simulink model "Quad_PID_attack_done"  (R2025a)
settings: Solver=ode4  StartTime=0.0  StopTime=40  FixedStep=0.001  RelTol=1e-3
undefined symbols (not defined in the file): DiscIntNeverNeededParam, Ts
libraries: simulink x6
settings Model: Creator=Qi  LastModifiedBy=shaoc
settings SolverCC: AlgebraicLoopSolver=TrustRegion
settings DataIOCC: ReturnWorkspaceOutputs=off
settings DebuggingCC: UnconnectedInputMsg=warning  UnconnectedOutputMsg=warning  UnconnectedLineMsg=warning  ArithmeticOperatorsInVariantConditions=warning
settings ModelReferenceCC: EnableRefExpFcnMdlSchedulingChecks=on
settings SFSimCC: CustomCodeUndefinedFunction=UseInterfaceOnly
settings RTWCC: GPUComputeCapability=3.5

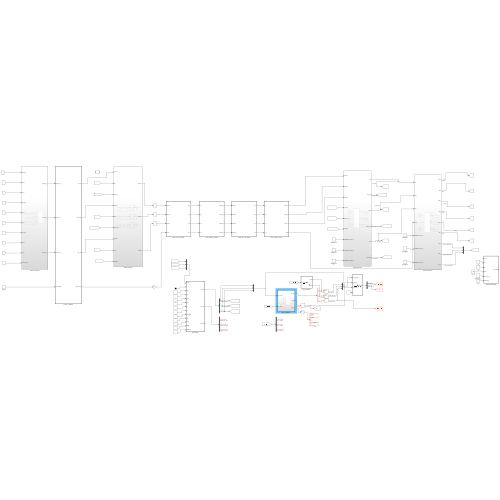
[thumbnail: Simulink's stored preview of the top-level diagram]
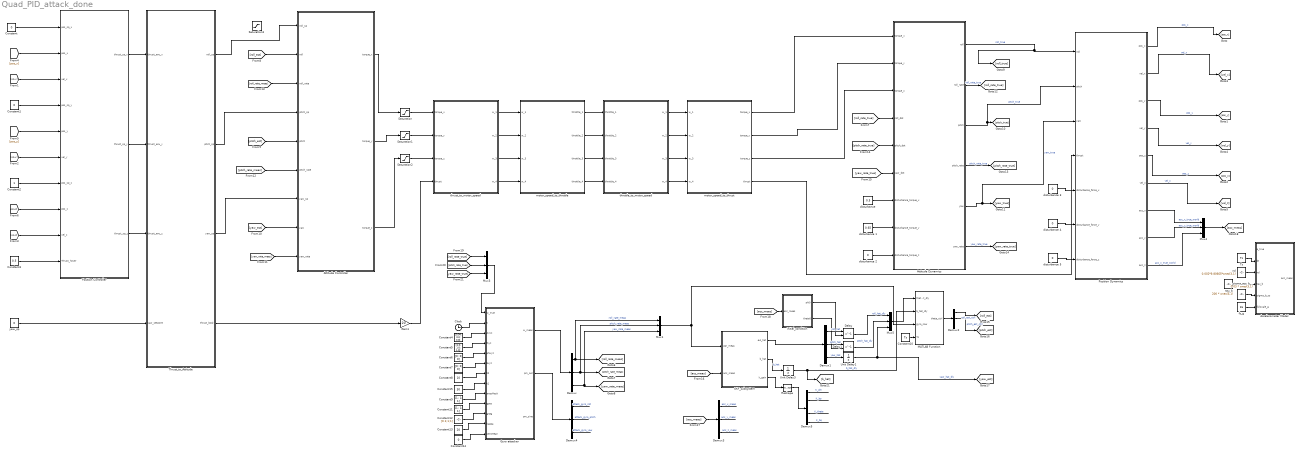
== system Quad_PID_attack_done ==
  Accelerometer Model : MATLAB Function  TreatAsAtomicUnit=on
  Attitude Controller : Subsystem
  Attitude Dynamics : Subsystem
  Clock : Clock
  Constant : Constant  Value=0
  Constant1 : Constant  Value=0
  Constant10 : Constant  Value=Ts  SampleTime=-1
  Constant11 : Constant  Value=[1; 1; 1]
  Constant12 : Constant  Value=[0.1;1;1]
  Constant13 : Constant  Value=20
  Constant14 : Constant  Value=0
  Constant15 : Constant  Value=30
  Constant2 : Constant
  Constant3 : Constant  Value=0.5
  Constant4 : Constant  Value=[0.04; 0.0; 0.0]
  Constant5 : Constant  Value=[1.0; 1.0; 1.0]
  Constant6 : Constant  Value=[0; 0; 0]
  Constant7 : Constant  Value=[0; 0; 0]
  Constant8 : Constant  Value=10
  Constant9 : Constant  Value=[1; 1; 1]
  Delay : Delay  DelayLength=1  InitialConditionSource=Input port  SampleTime=Ts
      settings: InputPortMap=u0,p4
  Delay1 : Delay  DelayLength=1  InitialConditionSource=Input port  SampleTime=Ts
      settings: InputPortMap=u0,p4
  Demux{,1..4} (5 alike) : Demux  Outputs=3
  Demux5 : Demux  Outputs=8
  EKF_subsystem : Subsystem  TreatAsAtomicUnit=on  SystemSampleTime=Ts
  Gain1 : Gain  Gain=20
  Gyro attacker : MATLAB Function  TreatAsAtomicUnit=on
  MATLAB Function : MATLAB Function  TreatAsAtomicUnit=on
  Mux{1,3..5} (4 alike) : Mux  Inputs=3
  Position Controller : Subsystem
  Position Dynamics : Subsystem
  Reshape : Reshape
  Saturation : Saturate  UpperLimit=1  LowerLimit=-1
  Saturation1 : Saturate  UpperLimit=1  LowerLimit=-1
  Saturation2 : Saturate  UpperLimit=1  LowerLimit=-1
  Saturation3 : Saturate  UpperLimit=10/180*pi  LowerLimit=-10/180*pi
  Thrust_to_Attitude : MATLAB Function  TreatAsAtomicUnit=on
  Ts : Constant  Value=Ts
  Unit Delay1 : UnitDelay  InitialCondition=true  SampleTime=Ts  HasFrameUpgradeWarning=on
  Unit Delay3 : UnitDelay  InitialCondition=true  SampleTime=Ts  HasFrameUpgradeWarning=on
  "disturbance " : Constant  Value=0.5
  disturbance 1 : Constant  Value=0.65
  disturbance {2..5} (4 alike) : Constant  Value=0
  "fs_g " : Constant  Value=16
  initial_condition : MATLAB Function  TreatAsAtomicUnit=on
  "motor_speed_to_throttle " : MATLAB Function  TreatAsAtomicUnit=on
  motor_speed_to_thrust : MATLAB Function  TreatAsAtomicUnit=on
  nd : Constant  Value=0.002*9.80665*ones(3,1)  VectorParams1D=off  LockScale=on
  sigma_acc_b : Constant  Value=0.03 * ones(3,1)  VectorParams1D=off  LockScale=on
  tau_b : Constant  Value=200 * ones(3,1)  VectorParams1D=off  LockScale=on
  throttle_to_motor_speed : MATLAB Function  TreatAsAtomicUnit=on
  thrust_to_motor_speed : MATLAB Function  TreatAsAtomicUnit=on
  yaw_sp : Constant  Value=0
  wires:
  yaw_sp/1 -> Thrust_to_Attitude/4(yaw_setpoint)
  Thrust_to_Attitude/4(thrust_body) -> Gain1/1
  Constant/1 -> Position Controller/1(pos_sp_x)
  [pos_x] -> Position Controller/2(pos_x)
  Constant1/1 -> Position Controller/4(pos_sp_y)
  [pos_z] -> Position Controller/8(pos_z)
  Constant2/1 -> Position Controller/7(pos_sp_z)
  Position Controller/1(thrust_sp_x) -> Thrust_to_Attitude/1(thrust_enu_x)
  Position Controller/2(thrust_sp_y) -> Thrust_to_Attitude/2(thrust_enu_y)
  Position Controller/3(thrust_sp_z) -> Thrust_to_Attitude/3(thrust_enu_z)
  [yaw_est] -> Attitude Controller/8(yaw)
  [roll_est] -> Attitude Controller/2(roll)
  [pitch_est] -> Attitude Controller/5(pitch)
  Thrust_to_Attitude/2(pitch_sp) -> Attitude Controller/4(pitch_sp)
  Thrust_to_Attitude/3(yaw_sp) -> Attitude Controller/7(yaw_sp)
  Attitude Controller/2(torque_y) -> Saturation1/1
  Attitude Controller/1(torque_x) -> Saturation/1
  Attitude Controller/3(torque_z) -> Saturation2/1
  [vel_x] -> Position Controller/3(vel_x)
  [pos_y] -> Position Controller/5(pos_y)
  [vel_y] -> Position Controller/6(vel_y)
  [vel_z] -> Position Controller/9(vel_z)
  [roll_rate_meas] -> Attitude Controller/3(roll_rate)
  [pitch_rate_meas] -> Attitude Controller/6(pitch_rate)
  [yaw_rate_meas] -> Attitude Controller/9(yaw_rate)
  Attitude Dynamics/3(pitch) -> Position Dynamics/2(pitch), [pitch_true]  "pitch_true"
  Attitude Dynamics/1(roll) -> [roll_true], Position Dynamics/1(roll)  "roll_true"
  Attitude Dynamics/5(yaw) -> [yaw_true], Position Dynamics/3(yaw)  "yaw_true"
  motor_speed_to_thrust/1(torque_x) -> Attitude Dynamics/1(torque_x)
  motor_speed_to_thrust/2(torque_y) -> Attitude Dynamics/2(torque_y)
  [roll_rate_true] -> Attitude Dynamics/4(roll_dot)
  motor_speed_to_thrust/3(torque_z) -> Attitude Dynamics/3(torque_z)
  [pitch_rate_true] -> Attitude Dynamics/5(pitch_dot)
  [yaw_rate_true] -> Attitude Dynamics/6(yaw_dot)
  Attitude Dynamics/2(roll_rate) -> [roll_rate_true]  "roll_rate_true"
  Attitude Dynamics/4(pitch_rate) -> [pitch_rate_true]  "pitch_rate_true"
  Attitude Dynamics/6(yaw_rate) -> [yaw_rate_true]  "yaw_rate_true"
  motor_speed_to_thrust/4(thrust) -> Position Dynamics/4(thrust)
  Position Dynamics/1(pos_x) -> [pos_x]  "pos_x"
  Position Dynamics/3(pos_y) -> [pos_y]  "pos_y"
  Position Dynamics/4(vel_y) -> [vel_y]  "vel_y"
  Position Dynamics/5(pos_z) -> [pos_z]  "pos_z"
  Position Dynamics/6(vel_z) -> [vel_z]  "vel_z"
  Constant3/1 -> Position Controller/10(Thrust_hover)
  disturbance 2/1 -> Attitude Dynamics/9(disturbance_torque_z)
  disturbance 1/1 -> Attitude Dynamics/8(disturbance_torque_y)
  "disturbance "/1 -> Attitude Dynamics/7(disturbance_torque_x)
  disturbance 3/1 -> Position Dynamics/5(disturbance_force_x)
  disturbance 4/1 -> Position Dynamics/6(disturbance_force_y)
  disturbance 5/1 -> Position Dynamics/7(disturbance_force_z)
  thrust_to_motor_speed/1(w_1) -> "motor_speed_to_throttle "/1(w_1)
  thrust_to_motor_speed/3(w_3) -> "motor_speed_to_throttle "/3(w_3)
  thrust_to_motor_speed/4(w_4) -> "motor_speed_to_throttle "/4(w_4)
  thrust_to_motor_speed/2(w_2) -> "motor_speed_to_throttle "/2(w_2)
  "motor_speed_to_throttle "/1(throttle_1) -> throttle_to_motor_speed/1(throttle_1)
  "motor_speed_to_throttle "/2(throttle_2) -> throttle_to_motor_speed/2(throttle_2)
  "motor_speed_to_throttle "/3(throttle_3) -> throttle_to_motor_speed/3(throttle_3)
  "motor_speed_to_throttle "/4(throttle_4) -> throttle_to_motor_speed/4(throttle_4)
  throttle_to_motor_speed/1(w_1) -> motor_speed_to_thrust/1(w_1)
  throttle_to_motor_speed/2(w_2) -> motor_speed_to_thrust/2(w_2)
  throttle_to_motor_speed/3(w_3) -> motor_speed_to_thrust/3(w_3)
  throttle_to_motor_speed/4(w_4) -> motor_speed_to_thrust/4(w_4)
  Gain1/1 -> thrust_to_motor_speed/4(thrust)
  Position Dynamics/2(vel_x) -> [vel_x]  "vel_x"
  Saturation/1 -> thrust_to_motor_speed/1(torque_x)
  Saturation1/1 -> thrust_to_motor_speed/2(torque_y)
  Saturation2/1 -> thrust_to_motor_speed/3(torque_z)
  Clock/1 -> Gyro attacker/2(t)
  Constant4/1 -> Gyro attacker/3(Axyz)
  Constant5/1 -> Gyro attacker/4(fxyz)
  Constant6/1 -> Gyro attacker/5(phixyz)
  Constant7/1 -> Gyro attacker/6(bxyz)
  Constant8/1 -> Gyro attacker/7(t0)
  Constant9/1 -> Gyro attacker/9(axesMask)
  Gyro attacker/1(w_meas) -> Demux/1
  Demux/1 -> Mux1/1, [roll_rate_meas]  "roll_rate_meas"
  Demux/2 -> Mux1/2, [pitch_rate_meas]  "pitch_rate_meas"
  Demux/3 -> Mux1/3, [yaw_rate_meas]  "yaw_rate_meas"
  Position Dynamics/7(acc_x) -> Mux4/1  "acc_x_true_world"
  Position Dynamics/8(acc_y) -> Mux4/2  "acc_y_true_world"
  Position Dynamics/9(acc_z) -> Mux4/3  "acc_z_true_world"
  [roll_rate_true] -> Mux3/1
  [pitch_rate_true] -> Mux3/2
  [yaw_rate_true] -> Mux3/3
  Mux3/1 -> Gyro attacker/1(w_true)
  Mux1/1 -> MATLAB Function/3(gyro_now), EKF_subsystem/1(pqr_meas)
  EKF_subsystem/1(eul_hat) -> Demux1/1
  Demux1/1 -> Delay/1  "roll_hat"
  Delay/1 -> Mux5/1  "roll_hat_dly"
  Demux1/2 -> Delay1/1  "pitch_hat"
  Delay1/1 -> Mux5/2  "pitch_hat_dly"
  Demux1/3 -> Unit Delay1/1  "yaw_hat"
  Unit Delay1/1 -> Mux5/3, [yaw_est]  "yaw_hat_dly"
  EKF_subsystem/2(b_hat) -> Unit Delay3/1  "b_hat"
  Unit Delay3/1 -> MATLAB Function/2(b_hat_dly), [b_hat]  "b_hat_dly"
  Mux5/1 -> MATLAB Function/1(theta_hat_dly)
  Constant10/1 -> MATLAB Function/4(Ts)
  MATLAB Function/1(theta_ctrl) -> Demux2/1
  Demux2/1 -> [roll_est]  "roll_est_ctrl"
  Demux2/2 -> [pitch_est]  "pitch_est_ctrl"
  [acc_meas] -> EKF_subsystem/2(acc_meas)
  [acc_meas] -> Demux3/1
  Demux3/1 -> ?  "acc_x_meas"
  Demux3/2 -> ?  "acc_y_meas"
  Demux3/3 -> ?  "acc_z_meas"
  [acc_meas] -> initial_condition/1(acc_meas)
  initial_condition/1(phi0) -> Delay/2
  initial_condition/2(theta0) -> Delay1/2
  Ts/1 -> Accelerometer Model/2(dt)
  "fs_g "/1 -> Accelerometer Model/6(fullscale_g)
  nd/1 -> Accelerometer Model/3(nd)
  tau_b/1 -> Accelerometer Model/4(tau_b)
  sigma_acc_b/1 -> Accelerometer Model/5(sigma_b_ss)
  Mux4/1 -> [acc_meas]
  Demux4/3 -> ?  "attack_gyro_yaw"
  Demux4/1 -> ?  "attack_gyro_roll"
  Gyro attacker/2(pm_out) -> Demux4/1
  Demux4/2 -> ?  "attack_gyro_pitch"
  Constant11/1 -> Gyro attacker/10(gpos)
  Constant12/1 -> Gyro attacker/11(gneg)
  Constant13/1 -> Gyro attacker/12(kappa)
  Constant14/1 -> Gyro attacker/13(zeroMean)
  Constant15/1 -> Gyro attacker/8(t1)
  EKF_subsystem/3(k_gain) -> Reshape/1
  Reshape/1 -> Demux5/1
  Demux5/1 -> ?  "K_phi"
  Demux5/3 -> ?  "K_bp"
  Demux5/6 -> ?  "K_theta"
  Demux5/8 -> ?  "K_bq"
  Thrust_to_Attitude/1(roll_sp) -> Attitude Controller/1(roll_sp)

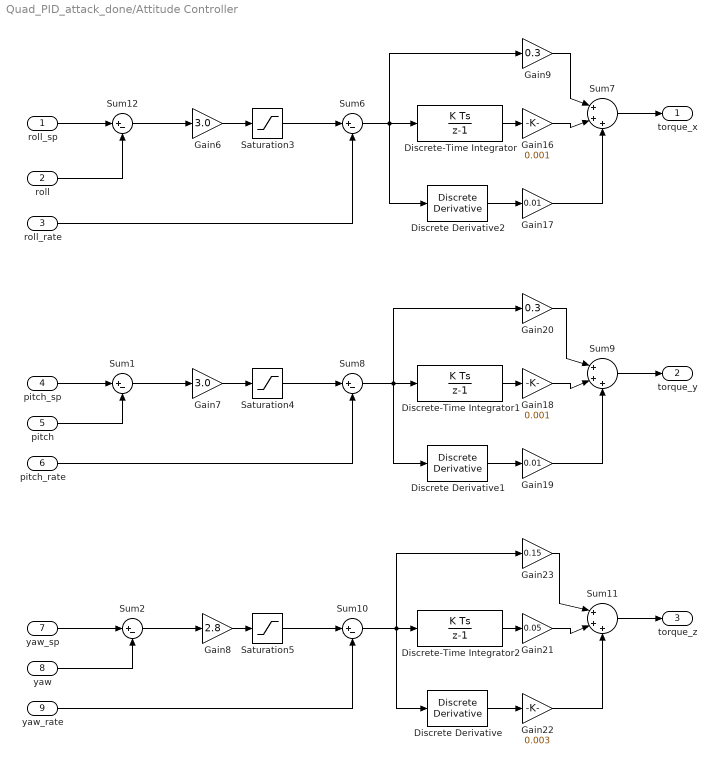
== system Quad_PID_attack_done/Attitude Controller ==
  roll_sp : Inport
  roll : Inport  Port=2
  roll_rate : Inport  Port=3
  pitch_sp : Inport  Port=4
  pitch : Inport  Port=5
  pitch_rate : Inport  Port=6
  yaw_sp : Inport  Port=7
  yaw : Inport  Port=8
  yaw_rate : Inport  Port=9
  Discrete Derivative : simulink/Discrete/Discrete Derivative  gainval=1.0  ICPrevScaledInput=0.0  OutMin=[]  OutMax=[]  OutDataType=fixdt(1, 16)  OutScaling=2^-10  DoSatur=off
  Discrete Derivative1 : simulink/Discrete/Discrete Derivative  gainval=1.0  ICPrevScaledInput=0.0  OutMin=[]  OutMax=[]  OutDataType=fixdt(1, 16)  OutScaling=2^-10  DoSatur=off
  Discrete Derivative2 : simulink/Discrete/Discrete Derivative  gainval=1.0  ICPrevScaledInput=0.0  OutMin=[]  OutMax=[]  OutDataType=fixdt(1, 16)  OutScaling=2^-10  DoSatur=off
  Discrete-Time Integrator : DiscreteIntegrator  SampleTime=-1  LimitOutput=on  UpperSaturationLimit=0.3  LowerSaturationLimit=-0.3  ICPrevOutput=DiscIntNeverNeededParam  ICPrevScaledInput=DiscIntNeverNeededParam
  Discrete-Time Integrator1 : DiscreteIntegrator  SampleTime=-1  LimitOutput=on  UpperSaturationLimit=0.3  LowerSaturationLimit=-0.3  ICPrevOutput=DiscIntNeverNeededParam  ICPrevScaledInput=DiscIntNeverNeededParam
  Discrete-Time Integrator2 : DiscreteIntegrator  SampleTime=-1  LimitOutput=on  UpperSaturationLimit=0.3  LowerSaturationLimit=-0.3  ICPrevOutput=DiscIntNeverNeededParam  ICPrevScaledInput=DiscIntNeverNeededParam
  Gain16 : Gain  Gain=0.001
  Gain17 : Gain  Gain=0.01
  Gain18 : Gain  Gain=0.001
  Gain19 : Gain  Gain=0.01
  Gain20 : Gain  Gain=0.3
  Gain21 : Gain  Gain=0.05
  Gain22 : Gain  Gain=0.003
  Gain23 : Gain  Gain=0.15
  Gain6 : Gain  Gain=3.0
  Gain7 : Gain  Gain=3.0
  Gain8 : Gain  Gain=2.8
  Gain9 : Gain  Gain=0.3
  Saturation3 : Saturate  UpperLimit=220/180*pi  LowerLimit=-220/180*pi
  Saturation4 : Saturate  UpperLimit=220/180*pi  LowerLimit=-220/180*pi
  Saturation5 : Saturate  UpperLimit=220/180*pi  LowerLimit=-220/180*pi
  Sum{1..2,6,8,10,12} (6 alike) : Sum  Inputs=|+-
  Sum11 : Sum  Inputs=|+++
  Sum7 : Sum  Inputs=|+++
  Sum9 : Sum  Inputs=|+++
  torque_x : Outport  VectorParamsAs1DForOutWhenUnconnected=off
  torque_y : Outport  Port=2  VectorParamsAs1DForOutWhenUnconnected=off
  torque_z : Outport  Port=3  VectorParamsAs1DForOutWhenUnconnected=off
  wires:
  Gain8/1 -> Saturation5/1
  Sum10/1 -> Discrete-Time Integrator2/1, Discrete Derivative/1, Gain23/1
  Sum6/1 -> Discrete-Time Integrator/1, Discrete Derivative2/1, Gain9/1
  Saturation4/1 -> Sum8/1
  Sum7/1 -> torque_x/1
  Discrete-Time Integrator2/1 -> Gain21/1
  Gain16/1 -> Sum7/2
  Sum8/1 -> Discrete-Time Integrator1/1, Discrete Derivative1/1, Gain20/1
  yaw_rate/1 -> Sum10/2
  Saturation5/1 -> Sum10/1
  Gain23/1 -> Sum11/1
  Saturation3/1 -> Sum6/1
  Discrete Derivative1/1 -> Gain19/1
  Gain17/1 -> Sum7/3
  Gain19/1 -> Sum9/3
  Gain22/1 -> Sum11/3
  Discrete Derivative/1 -> Gain22/1
  Gain7/1 -> Saturation4/1
  Discrete-Time Integrator1/1 -> Gain18/1
  Gain18/1 -> Sum9/2
  Gain9/1 -> Sum7/1
  Gain20/1 -> Sum9/1
  Discrete-Time Integrator/1 -> Gain16/1
  roll_rate/1 -> Sum6/2
  Sum9/1 -> torque_y/1
  Discrete Derivative2/1 -> Gain17/1
  Gain21/1 -> Sum11/2
  Gain6/1 -> Saturation3/1
  Sum11/1 -> torque_z/1
  pitch_rate/1 -> Sum8/2
  yaw/1 -> Sum2/2
  Sum1/1 -> Gain7/1
  roll_sp/1 -> Sum12/1
  pitch/1 -> Sum1/2
  Sum2/1 -> Gain8/1
  pitch_sp/1 -> Sum1/1
  roll/1 -> Sum12/2
  yaw_sp/1 -> Sum2/1
  Sum12/1 -> Gain6/1

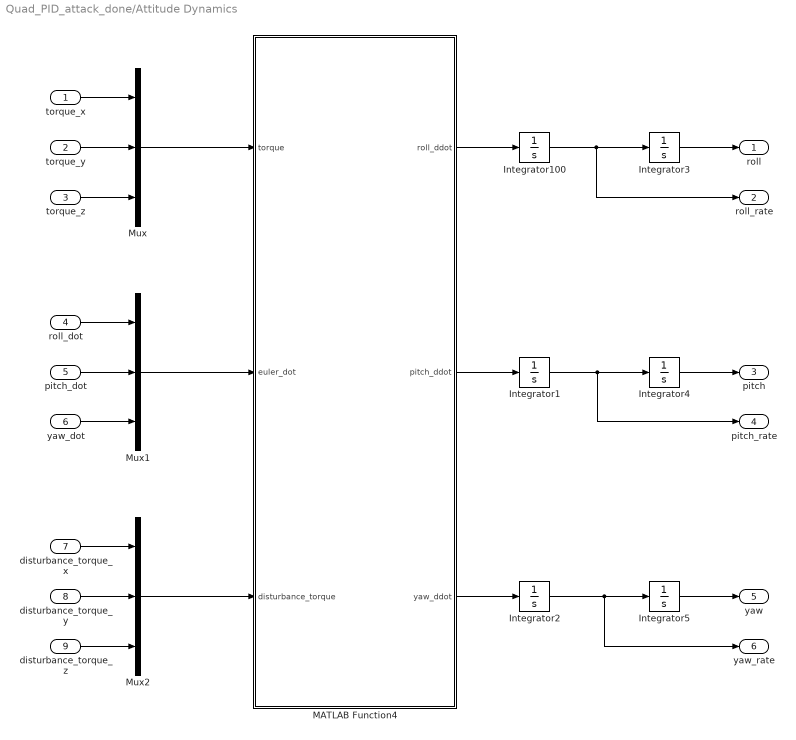
== system Quad_PID_attack_done/Attitude Dynamics ==
  torque_x : Inport
  torque_y : Inport  Port=2
  torque_z : Inport  Port=3
  roll_dot : Inport  Port=4
  pitch_dot : Inport  Port=5
  yaw_dot : Inport  Port=6
  disturbance_torque_x : Inport  Port=7
  disturbance_torque_y : Inport  Port=8
  disturbance_torque_z : Inport  Port=9
  Integrator{1..5,100} (6 alike) : Integrator
  MATLAB Function4 : MATLAB Function  TreatAsAtomicUnit=on
  Mux : Mux  Inputs=3
  Mux1 : Mux  Inputs=3
  Mux2 : Mux  Inputs=3
  roll : Outport  VectorParamsAs1DForOutWhenUnconnected=off
  roll_rate : Outport  Port=2  VectorParamsAs1DForOutWhenUnconnected=off
  pitch : Outport  Port=3  VectorParamsAs1DForOutWhenUnconnected=off
  pitch_rate : Outport  Port=4  VectorParamsAs1DForOutWhenUnconnected=off
  yaw : Outport  Port=5  VectorParamsAs1DForOutWhenUnconnected=off
  yaw_rate : Outport  Port=6  VectorParamsAs1DForOutWhenUnconnected=off
  wires:
  Integrator100/1 -> roll_rate/1, Integrator3/1
  Integrator4/1 -> pitch/1
  MATLAB Function4/3(yaw_ddot) -> Integrator2/1
  Integrator3/1 -> roll/1
  Integrator1/1 -> pitch_rate/1, Integrator4/1
  Integrator2/1 -> yaw_rate/1, Integrator5/1
  MATLAB Function4/1(roll_ddot) -> Integrator100/1
  MATLAB Function4/2(pitch_ddot) -> Integrator1/1
  Integrator5/1 -> yaw/1
  disturbance_torque_y/1 -> Mux2/2
  disturbance_torque_z/1 -> Mux2/3
  disturbance_torque_x/1 -> Mux2/1
  Mux2/1 -> MATLAB Function4/3(disturbance_torque)
  yaw_dot/1 -> Mux1/3
  pitch_dot/1 -> Mux1/2
  roll_dot/1 -> Mux1/1
  Mux1/1 -> MATLAB Function4/2(euler_dot)
  torque_y/1 -> Mux/2
  torque_z/1 -> Mux/3
  torque_x/1 -> Mux/1
  Mux/1 -> MATLAB Function4/1(torque)

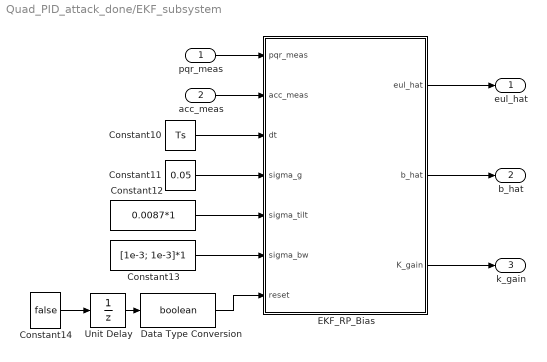
== system Quad_PID_attack_done/EKF_subsystem ==
  pqr_meas : Inport
  acc_meas : Inport  Port=2
  Constant10 : Constant  Value=Ts  SampleTime=-1
  Constant11 : Constant  Value=0.05
  Constant12 : Constant  Value=0.0087*1
  Constant13 : Constant  Value=[1e-3; 1e-3]*1
  Constant14 : Constant  Value=false
  Data Type Conversion : DataTypeConversion  OutDataTypeStr=boolean  SaturateOnIntegerOverflow=off  RndMeth=Floor
  EKF_RP_Bias : MATLAB Function  TreatAsAtomicUnit=on
  Unit Delay : UnitDelay  InitialCondition=true  SampleTime=Ts  HasFrameUpgradeWarning=on
  eul_hat : Outport  VectorParamsAs1DForOutWhenUnconnected=off
  b_hat : Outport  Port=2  VectorParamsAs1DForOutWhenUnconnected=off
  k_gain : Outport  Port=3  VectorParamsAs1DForOutWhenUnconnected=off
  wires:
  Unit Delay/1 -> Data Type Conversion/1
  Constant14/1 -> Unit Delay/1
  Constant11/1 -> EKF_RP_Bias/4(sigma_g)
  Constant10/1 -> EKF_RP_Bias/3(dt)
  Data Type Conversion/1 -> EKF_RP_Bias/7(reset)
  Constant13/1 -> EKF_RP_Bias/6(sigma_bw)
  Constant12/1 -> EKF_RP_Bias/5(sigma_tilt)
  EKF_RP_Bias/1(eul_hat) -> eul_hat/1
  EKF_RP_Bias/2(b_hat) -> b_hat/1
  pqr_meas/1 -> EKF_RP_Bias/1(pqr_meas)
  acc_meas/1 -> EKF_RP_Bias/2(acc_meas)
  EKF_RP_Bias/3(K_gain) -> k_gain/1

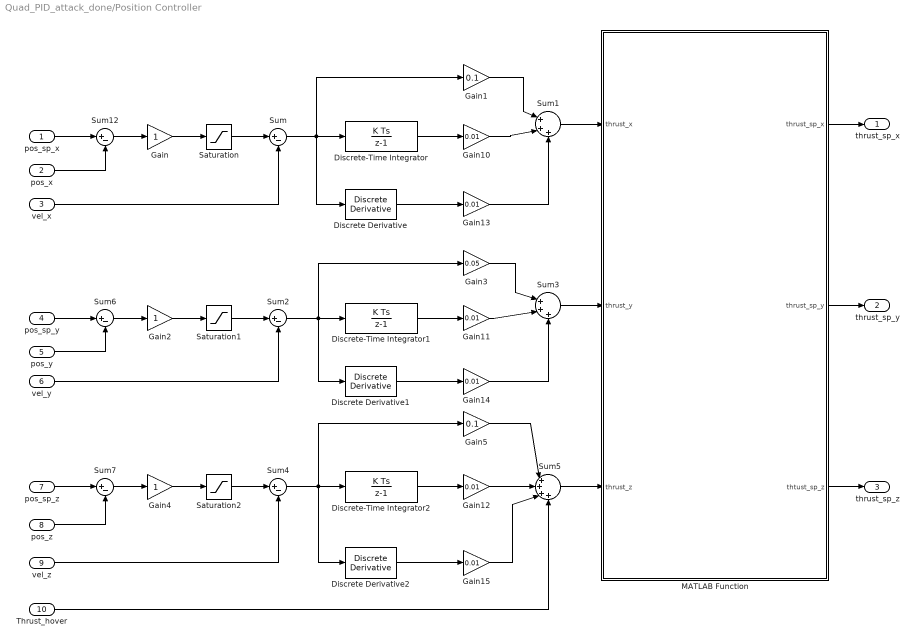
== system Quad_PID_attack_done/Position Controller ==
  pos_sp_x : Inport
  pos_x : Inport  Port=2
  vel_x : Inport  Port=3
  pos_sp_y : Inport  Port=4
  pos_y : Inport  Port=5
  vel_y : Inport  Port=6
  pos_sp_z : Inport  Port=7
  pos_z : Inport  Port=8
  vel_z : Inport  Port=9
  Thrust_hover : Inport  Port=10
  Discrete Derivative : simulink/Discrete/Discrete Derivative  gainval=1.0  ICPrevScaledInput=0.0  OutMin=[]  OutMax=[]  OutDataType=fixdt(1, 16)  OutScaling=2^-10  DoSatur=off
  Discrete Derivative1 : simulink/Discrete/Discrete Derivative  gainval=1.0  ICPrevScaledInput=0.0  OutMin=[]  OutMax=[]  OutDataType=fixdt(1, 16)  OutScaling=2^-10  DoSatur=off
  Discrete Derivative2 : simulink/Discrete/Discrete Derivative  gainval=1.0  ICPrevScaledInput=0.0  OutMin=[]  OutMax=[]  OutDataType=fixdt(1, 16)  OutScaling=2^-10  DoSatur=off
  Discrete-Time Integrator : DiscreteIntegrator  SampleTime=-1  LimitOutput=on  UpperSaturationLimit=0.9  LowerSaturationLimit=-0.9  ICPrevOutput=DiscIntNeverNeededParam  ICPrevScaledInput=DiscIntNeverNeededParam
  Discrete-Time Integrator1 : DiscreteIntegrator  SampleTime=-1  LimitOutput=on  UpperSaturationLimit=0.9  LowerSaturationLimit=-0.9  ICPrevOutput=DiscIntNeverNeededParam  ICPrevScaledInput=DiscIntNeverNeededParam
  Discrete-Time Integrator2 : DiscreteIntegrator  SampleTime=-1  LimitOutput=on  UpperSaturationLimit=0.9  LowerSaturationLimit=-0.9  ICPrevOutput=DiscIntNeverNeededParam  ICPrevScaledInput=DiscIntNeverNeededParam
  Gain : Gain
  Gain1 : Gain  Gain=0.1
  Gain{10..15} (6 alike) : Gain  Gain=0.01
  Gain2 : Gain
  Gain3 : Gain  Gain=0.05
  Gain4 : Gain
  Gain5 : Gain  Gain=0.1
  MATLAB Function : MATLAB Function  TreatAsAtomicUnit=on
  Saturation : Saturate  UpperLimit=5  LowerLimit=-5
  Saturation1 : Saturate  UpperLimit=5  LowerLimit=-5
  Saturation2 : Saturate  UpperLimit=2  LowerLimit=-2
  Sum{,2,4,6..7,12} (6 alike) : Sum  Inputs=|+-
  Sum1 : Sum  Inputs=|+++
  Sum3 : Sum  Inputs=|+++
  Sum5 : Sum  Inputs=|++++
  thrust_sp_x : Outport  VectorParamsAs1DForOutWhenUnconnected=off
  thrust_sp_y : Outport  Port=2  VectorParamsAs1DForOutWhenUnconnected=off
  thrust_sp_z : Outport  Port=3  VectorParamsAs1DForOutWhenUnconnected=off
  wires:
  Gain4/1 -> Saturation2/1
  Saturation1/1 -> Sum2/1
  MATLAB Function/1(thrust_sp_x) -> thrust_sp_x/1
  vel_x/1 -> Sum/2
  Gain/1 -> Saturation/1
  Gain11/1 -> Sum3/2
  Sum2/1 -> Discrete-Time Integrator1/1, Discrete Derivative1/1, Gain3/1
  Gain3/1 -> Sum3/1
  Sum4/1 -> Discrete-Time Integrator2/1, Discrete Derivative2/1, Gain5/1
  vel_z/1 -> Sum4/2
  Gain2/1 -> Saturation1/1
  Sum5/1 -> MATLAB Function/3(thrust_z)
  Discrete Derivative2/1 -> Gain15/1
  Saturation2/1 -> Sum4/1
  Discrete-Time Integrator/1 -> Gain10/1
  MATLAB Function/2(thrust_sp_y) -> thrust_sp_y/1
  MATLAB Function/3(thtust_sp_z) -> thrust_sp_z/1
  Saturation/1 -> Sum/1
  Gain1/1 -> Sum1/1
  Sum1/1 -> MATLAB Function/1(thrust_x)
  Gain13/1 -> Sum1/3
  Sum/1 -> Discrete-Time Integrator/1, Discrete Derivative/1, Gain1/1
  Discrete Derivative1/1 -> Gain14/1
  Discrete Derivative/1 -> Gain13/1
  Discrete-Time Integrator2/1 -> Gain12/1
  Discrete-Time Integrator1/1 -> Gain11/1
  Thrust_hover/1 -> Sum5/4
  Gain5/1 -> Sum5/1
  Sum3/1 -> MATLAB Function/2(thrust_y)
  Gain12/1 -> Sum5/2
  Gain15/1 -> Sum5/3
  Gain14/1 -> Sum3/3
  vel_y/1 -> Sum2/2
  pos_sp_x/1 -> Sum12/1
  Sum12/1 -> Gain/1
  pos_x/1 -> Sum12/2
  pos_sp_z/1 -> Sum7/1
  Sum7/1 -> Gain4/1
  pos_z/1 -> Sum7/2
  pos_y/1 -> Sum6/2
  Sum6/1 -> Gain2/1
  pos_sp_y/1 -> Sum6/1
  Gain10/1 -> Sum1/2

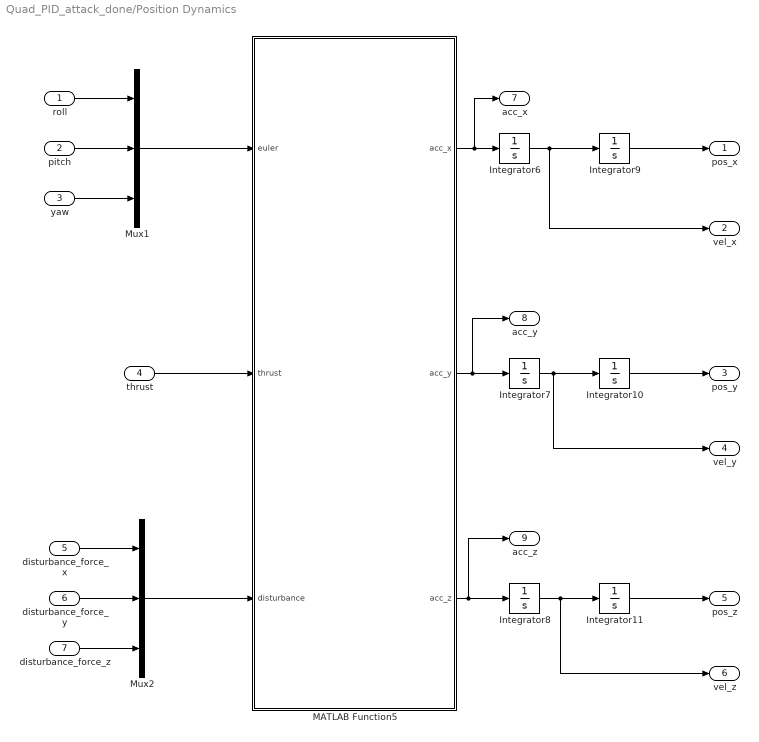
== system Quad_PID_attack_done/Position Dynamics ==
  roll : Inport
  pitch : Inport  Port=2
  yaw : Inport  Port=3
  thrust : Inport  Port=4
  disturbance_force_x : Inport  Port=5
  disturbance_force_y : Inport  Port=6
  disturbance_force_z : Inport  Port=7
  Integrator{6..11} (6 alike) : Integrator
  MATLAB Function5 : MATLAB Function  TreatAsAtomicUnit=on
  Mux1 : Mux  Inputs=3
  Mux2 : Mux  Inputs=3
  pos_x : Outport  VectorParamsAs1DForOutWhenUnconnected=off
  vel_x : Outport  Port=2  VectorParamsAs1DForOutWhenUnconnected=off
  pos_y : Outport  Port=3  VectorParamsAs1DForOutWhenUnconnected=off
  vel_y : Outport  Port=4  VectorParamsAs1DForOutWhenUnconnected=off
  pos_z : Outport  Port=5  VectorParamsAs1DForOutWhenUnconnected=off
  vel_z : Outport  Port=6  VectorParamsAs1DForOutWhenUnconnected=off
  acc_x : Outport  Port=7  VectorParamsAs1DForOutWhenUnconnected=off
  acc_y : Outport  Port=8  VectorParamsAs1DForOutWhenUnconnected=off
  acc_z : Outport  Port=9  VectorParamsAs1DForOutWhenUnconnected=off
  wires:
  Integrator7/1 -> vel_y/1, Integrator10/1
  MATLAB Function5/1(acc_x) -> acc_x/1, Integrator6/1
  MATLAB Function5/3(acc_z) -> acc_z/1, Integrator8/1
  Integrator6/1 -> vel_x/1, Integrator9/1
  MATLAB Function5/2(acc_y) -> acc_y/1, Integrator7/1
  thrust/1 -> MATLAB Function5/2(thrust)
  Integrator8/1 -> vel_z/1, Integrator11/1
  Integrator9/1 -> pos_x/1
  Integrator10/1 -> pos_y/1
  Integrator11/1 -> pos_z/1
  roll/1 -> Mux1/1
  pitch/1 -> Mux1/2
  Mux1/1 -> MATLAB Function5/1(euler)
  yaw/1 -> Mux1/3
  disturbance_force_x/1 -> Mux2/1
  disturbance_force_z/1 -> Mux2/3
  Mux2/1 -> MATLAB Function5/3(disturbance)
  disturbance_force_y/1 -> Mux2/2

== matlab function Quad_PID_attack_done/motor_speed_to_throttle  ==
  data: w_1 input; throttle_1 output; w_2 input; w_3 input; w_4 input; throttle_2 output; throttle_3 output; throttle_4 output
function [throttle_1, throttle_2, throttle_3, throttle_4] = motor_speed_to_throttle(w_1, w_2, w_3, w_4)
    %%注意转速单位 rad/s or rpm 转/分   
    k_est = 718.07;
    d_est = 88.448;
    
    throttle_1 = (w_1 - d_est)/k_est;
    throttle_2 = (w_2 - d_est)/k_est;
    throttle_3 = (w_3 - d_est)/k_est;
    throttle_4 = (w_4 - d_est)/k_est;
end

== matlab function Quad_PID_attack_done/throttle_to_motor_speed ==
  data: throttle_1 input; w_1 output; throttle_2 input; throttle_3 input; throttle_4 input; w_2 output; w_3 output; w_4 output
function [w_1, w_2, w_3, w_4] = throttle_tomotor_speed(throttle_1, throttle_2, throttle_3, throttle_4)
    k = 718.07;
    d = 88.448;
    
    w_1 = k * throttle_1 + d;
    w_2 = k * throttle_2 + d;
    w_3 = k * throttle_3 + d;
    w_4 = k * throttle_4 + d;
end

== matlab function Quad_PID_attack_done/motor_speed_to_thrust ==
  data: torque_x output; w_1 input; w_2 input; torque_y output; w_3 input; w_4 input; torque_z output; thrust output
function [torque_x, torque_y, torque_z, thrust] = thrust_to_motor_speed(w_1, w_2, w_3, w_4)

d  = 0.2;
cT = 1.239e-5;
cM = 1.982e-7;


M4 = [-sqrt(2)/2*d*cT,sqrt(2)/2*d*cT,sqrt(2)/2*d*cT,-sqrt(2)/2*d*cT;
       sqrt(2)/2*d*cT,-sqrt(2)/2*d*cT,sqrt(2)/2*d*cT,-sqrt(2)/2*d*cT;
       cM,cM,-cM,-cM;
       cT,cT,cT,cT;];
   
u = M4 * [w_1^2 ;w_2^2 ;w_3^2 ;w_4^2];  

torque_x = u(1);
torque_y = u(2);
torque_z = u(3);
thrust   = u(4);


end

== matlab function Quad_PID_attack_done/Gyro attacker ==
  data: w_true input double size=[3 1]; w_meas output double size=[3 1]; t input double size=[1 1]; Axyz input double size=[3 1]; fxyz input double size=[3 1]; phixyz input double size=[3 1]; bxyz input double size=[3 1]; t0 input double size=[1 1]; t1 input; axesMask input double size=[3 1]; pm_out output; gpos input; gneg input; kappa input; zeroMean input; pm_sine output
function [w_meas, pm_out, pm_sine] = gyro_attack_asym_smooth_stateless( ...
    w_true, t, Axyz, fxyz, phixyz, bxyz, t0, t1, axesMask, ...
    gpos, gneg, kappa, zeroMean)
%#codegen
% Smooth (differentiable) asymmetric sine attack WITHOUT persistent state.
% Attack (including bias) is ON only for t0 <= t < t1. Outside: no attack.

% ---- ensure 3x1 columns ----
w_true   = reshape(w_true,   3,1);
Axyz     = reshape(Axyz,     3,1);
fxyz     = reshape(fxyz,     3,1);
phixyz   = reshape(phixyz,   3,1);
bxyz     = reshape(bxyz,     3,1);
axesMask = reshape(axesMask, 3,1);
gpos     = reshape(gpos,     3,1);
gneg     = reshape(gneg,     3,1);

% ---- timing, mask, enable-window ----
win   = double( (t >= t0) && (t < t1) );   % <-- NEW: window gate
t_eff = max(t - t0, 0);                    % time since start (phase continuity)
mask  = double(axesMask ~= 0);

% ---- base sine ----
arg = 2*pi.*fxyz.*t_eff + phixyz;
s   = sin(arg);

% ---- smooth gate & shaping (C^inf) ----
H        = 0.5 * (1 + tanh(kappa * s));       % 0..1 smoothly across s=0
gain_s   = gneg + (gpos - gneg) .* H;         % per-axis, smooth
s_shaped = gain_s .* s;                       % unitless

% ---- optional analytic DC removal (approx) ----
% Hard half-wave has mean (gpos-gneg)/pi; for smooth gate this is close.
if zeroMean ~= 0
    s_shaped = s_shaped - (gpos - gneg)/pi;
end

% ---- scale by amplitude ----
pm_sine_nom = Axyz .* s_shaped;               % rad/s (sine-only)

% ---- add bias, apply mask & window ----
% (bias is included ONLY inside [t0, t1) as requested)
pm_nom  = bxyz + pm_sine_nom;                 % rad/s (bias + sine)
pm_out  = win * (mask .* pm_nom);             % zero outside window
pm_sine = win * (mask .* pm_sine_nom);        % zero outside window

% ---- attacked measurement ----
w_meas = w_true + pm_out;
end

== matlab function Quad_PID_attack_done/MATLAB Function ==
  data: theta_hat_dly input double size=[3 1]; theta_ctrl output double size=[3 1]; b_hat_dly input double size=[3 1]; gyro_now input double size=[3 1]; Ts input double size=[1 1]
function theta_ctrl = predict_angle(theta_hat_dly, b_hat_dly, gyro_now, Ts)
% theta_hat_d: [phi_hat_d; theta_hat_d; psi_hat_d]
% b_hat_d    : [b_phi_d; b_theta_d; b_psi_hat_d]
% gyro_now   : [p_now; q_now; r_now] (rad/s)
% Ts         : sample time (s)
% Output:
% theta_ctrl : [phi_ctrl; theta_ctrl, psi_ctrl]

theta_ctrl = theta_hat_dly + Ts*(gyro_now - b_hat_dly);
end

== matlab function Quad_PID_attack_done/Accelerometer Model ==
  data: a_true input; acc_meas output; dt input; nd input; tau_b input; sigma_b_ss input; fullscale_g input
function acc_meas = accel_px4_noise(a_true, dt, nd, tau_b, sigma_b_ss, fullscale_g)
%#codegen
% a_true      : 3x1 true specific force in BODY [m/s^2]
% dt          : sample time [s]
% nd          : 3x1 white-noise density [m/s^2/sqrt(Hz)]  (PX4 accel_noise_density)
% tau_b       : 3x1 bias correlation time constant [s]    (PX4 accel_bias_tau ~ 100..500 s)
% sigma_b_ss  : 3x1 steady-state bias std [m/s^2]         (PX4 accel_bias_sigma ~ few cm/s^2)
% fullscale_g : scalar full-scale in g for clipping (e.g., 16). Use <=0 to disable.
%
% Output:
% a_meas      : 3x1 noisy accelerometer measurement [m/s^2]
%
% Model:
%   White noise      n_k ~ N(0, sigma_w^2) with sigma_w = nd / sqrt(dt)
%   Bias (Gauss-Markov/1st order):
%       b_{k+1} = exp(-dt/tau_b) .* b_k + sigma_b_ss .* sqrt(1 - exp(-2dt/tau_b)) .* w_k
%   Clip to +/- fullscale_g * g if requested.
%
% Notes:
% - This expects ENU or NED *specific force* already in BODY; the frame doesn’t matter here.
% - Use the same dt as your IMU sample time.
% - Typical PX4-ish numbers (convert g to m/s^2 with g0 = 9.80665):
%       nd ≈ 0.002*g0 [m/s^2/sqrt(Hz)]  (good MEMS)
%       tau_b ≈ 200 [s]
%       sigma_b_ss ≈ 0.03 [m/s^2]       (~3 mg)
%
% Author: you :)

persistent b rng_was_seeded
if isempty(b)
    b = zeros(3,1,'like',a_true);   % start bias at 0 (or make it an input if you prefer)
    rng_was_seeded = false;
end

% (Optional) deterministic seed once if you want repeatability during codegen sim
if ~rng_was_seeded
    % rng(1);  % uncomment for repeatable runs in normal mode (ignored in codegen)
    rng_was_seeded = true;
end

% ----- White noise std from density -----
% For a sampled white process with noise density nd [unit/sqrt(Hz)],
% the discrete-time std is approximately nd / sqrt(dt).
sigma_w = nd ./ sqrt(max(dt, eps));   % 3x1

% ----- Bias: 1st-order Gauss-Markov (per axis) -----
% alpha = exp(-dt/tau), q = sigma_ss * sqrt(1 - alpha^2)
alpha = exp(-dt ./ max(tau_b, 1e-9));                 % avoid div-by-zero
q_b   = sigma_b_ss .* sqrt(max(1 - alpha.^2, 0));     % ensure non-negative inside sqrt

% update bias
b = alpha .* b + q_b .* [randn; randn; randn];

% ----- Compose measurement -----
acc_meas = a_true ...
         + b ...
         + sigma_w .* [randn; randn; randn];

% ----- Clip to full-scale if requested -----
if fullscale_g > 0
    g0 = 9.80665;
    fs = fullscale_g * g0;
    acc_meas = min(max(acc_meas, -fs), fs);
end
end

== matlab function Quad_PID_attack_done/initial_condition ==
  data: acc_meas input; phi0 output; theta0 output
function [phi0, theta0] = tilt_from_acc_ic(acc_meas)
% acc_meas: BODY specific force [ax; ay; az] (m/s^2), body-Z up.
% Use the same axis flips as in your EKF:
sX = 1;  % set to your EKF’s sX
sY = 1;  % set to your EKF’s sY
sZ = +1;  % set to your EKF’s sZ

ax = sX*acc_meas(1);
ay = sY*acc_meas(2);
az = sZ*acc_meas(3);

den = hypot(ay, az);
if den < 1e-6
   phi0 = 0; theta0 = 0;   % fallback if nearly singular
else
   phi0   = atan2(+ay, +az);     % roll from y/z (Z up)
   theta0 = atan2(-ax,  den);    % pitch from x & |yz|
end

== matlab function Quad_PID_attack_done/Thrust_to_Attitude ==
  data: thrust_enu_x input; roll_sp output; thrust_enu_y input; thrust_enu_z input; pitch_sp output; yaw_sp output; yaw_setpoint input; thrust_body output
function [roll_sp,pitch_sp, yaw_sp,thrust_body] = Thrust_to_Attitude(thrust_enu_x,thrust_enu_y,thrust_enu_z,yaw_setpoint)

    thrust_sp = [thrust_enu_x;thrust_enu_y;thrust_enu_z];

    yaw_sp = yaw_setpoint;
    
    thrust_sp_length = norm(thrust_sp);
    
    thrust_body = thrust_sp_length;

    if thrust_sp_length > 0.00001 
        body_z = thrust_sp/thrust_sp_length;
    else 
        body_z = [0;0;1];
    end
    
     y_C= [-sin(yaw_sp);cos(yaw_sp);0];

    if abs(body_z(3)) > 0.000001
        body_x = cross( y_C,body_z);
        if body_z(3) < 0.0 
           body_x = -body_x;
        end
        body_x = body_x/norm(body_x);
    else 
        body_x = [0;0;1];
    end
    
    body_y = cross( body_z,body_x);
    
    R_sp = [body_x,body_y,body_z];
    
    euler_sp = rotation_to_euler(R_sp);
    
    roll_sp  = euler_sp(1);
    pitch_sp = euler_sp(2);
    yaw_sp   = euler_sp(3);
end

function euler_angle = rotation_to_euler(dcm)

    euler_angle = zeros(3,1);
    phi_val = atan2(dcm(3, 2), dcm(3, 3));
    theta_val = asin(-dcm(3, 1));
    psi_val = atan2(dcm(2, 1), dcm(1, 1));

    if abs(theta_val - pi / 2.0) < 1.0e-3 
        phi_val = 0.0;
        psi_val = atan2(dcm(2, 3), dcm(1, 3));
    elseif abs(theta_val + pi / 2.0) <  1.0e-3
        phi_val = 0.0;
        psi_val = atan2(-dcm(2, 3), -dcm(1, 3));
    end

    euler_angle(1) = phi_val;
    euler_angle(2) = theta_val;
    euler_angle(3) = psi_val;

end

== matlab function Quad_PID_attack_done/Position Controller/MATLAB Function ==
  data: thrust_x input; thrust_sp_x output; thrust_y input; thrust_z input; thrust_sp_y output; thtust_sp_z output
function [thrust_sp_x,thrust_sp_y,thtust_sp_z] = Thrust_Limit(thrust_x,thrust_y,thrust_z)

MPC_THR_MIN = 0.1;
MPC_THR_MAX = 0.9;
tilt_max = 20;

thtust_sp_z = constrain_function2( thrust_z, MPC_THR_MIN, MPC_THR_MAX);

thrust_max_XY_tilt = abs(thtust_sp_z) * tan(tilt_max/180.0*pi);
thrust_max_XY = sqrt(MPC_THR_MAX * MPC_THR_MAX - thtust_sp_z * thtust_sp_z);

thrust_max_XY = min(thrust_max_XY_tilt, thrust_max_XY);


if (thrust_x^2 + thrust_y^2) > thrust_max_XY^2 
    mag = sqrt(thrust_x^2 + thrust_y^2);
    thrust_sp_x = thrust_x / mag * thrust_max_XY;
    thrust_sp_y = thrust_y / mag * thrust_max_XY;
else
    thrust_sp_x = thrust_x;
    thrust_sp_y = thrust_y;
end

end
function output = constrain_function2(data, Min, Max)
    
    if data > Max
        output =  Max;
    elseif data < Min
        output = Min;
    else
        output = data;
    end
end

== matlab function Quad_PID_attack_done/thrust_to_motor_speed ==
  data: w_1 output; torque_x input; torque_y input; w_2 output; torque_z input; thrust input; w_3 output; w_4 output
function [w_1, w_2, w_3, w_4] = thrust_to_motor_speed(torque_x, torque_y, torque_z, thrust)
% Convert desired body torques + total thrust into rotor speeds for an X quad.
% Robust to infeasible mixes (prevents sqrt of negative).

% --- Parameters (tune to your vehicle) ---
d       = 0.20;          % [m] half-arm length (distance from CoM to rotor)
cT_est  = 1.239e-5;      % [N/(rad/s)^2] thrust coeff
cM_est  = 1.982e-7;      % [N·m/(rad/s)^2] yaw moment coeff (drag)
w_min   = 0.0;           % [rad/s] rotor min speed (0 if you allow stop)
w_max   = 2000.0;        % [rad/s] rotor max speed (example)

% Protect coefficients
cT = max(cT_est, eps);
cM = max(cM_est, eps);

% --- Allocation matrix (maps omega^2 -> [tau_x; tau_y; tau_z; Thrust]) ---
% X configuration, order motors [1..4] around the frame.
k = sqrt(2)/2*d*cT;
M4 = [ -k,  +k,  +k,  -k;           % tau_x
       +k,  -k,  +k,  -k;           % tau_y
       +cM, +cM, -cM, -cM;          % tau_z (CW/CW/CCW/CCW assumption)
       +cT, +cT, +cT, +cT ];        % Thrust

b  = [torque_x; torque_y; torque_z; thrust];

% --- Solve for omega^2 (can be negative if infeasible/noisy) ---
omega2 = M4 \ b;                     % 4x1

% Make sure it is real and finite
omega2(~isfinite(omega2)) = 0;
omega2 = real(omega2);

% --- Enforce non-negativity before sqrt ---
omega2 = max(omega2, 0);

% --- Recenter with an equal offset to match total thrust exactly ---
% We want cT*sum(omega2) == thrust  => add a common delta to each omega2
sum_now = cT*sum(omega2);
delta   = (thrust - sum_now)/(4*cT);     % common offset in omega^2 domain
omega2  = omega2 + delta;

% Re-clip negatives (if offset pushed some below zero)
omega2 = max(omega2, 0);

% --- If still not matching thrust (due to clipping), rescale positives ---
sum_now = cT*sum(omega2);
if sum_now > 0
    scale  = thrust / sum_now;
    omega2 = omega2 * scale;
else
    % If everything zero (thrust <= 0 after clipping), keep zeros
    omega2 = zeros(4,1);
end

% --- Saturate to physical speed limits (in omega^2 domain) ---
omega2_min = (w_min)^2;
omega2_max = (w_max)^2;
omega2 = min(max(omega2, omega2_min), omega2_max);

% --- Final rotor speeds ---
w = sqrt(omega2);

w_1 = w(1);
w_2 = w(2);
w_3 = w(3);
w_4 = w(4);
end

== matlab function Quad_PID_attack_done/EKF_subsystem/EKF_RP_Bias ==
  data: pqr_meas input double size=[3 1]; eul_hat output double size=[3 1]; acc_meas input double size=[3 1]; dt input double size=[1 1]; sigma_g input double size=[1 1]; sigma_tilt input double size=[1 1]; sigma_bw input double size=[2 1]; reset input boolean size=[1 1]; b_hat output double size=[3 1]; K_gain output
function [eul_hat, b_hat, K_gain] = EKF_RP_Bias(pqr_meas, acc_meas, dt, ...
                                        sigma_g, sigma_tilt, sigma_bw, reset)
% Roll–pitch EKF with gyro bias on p,q. Yaw dead-reckoned.
% x = [phi; theta; bp; bq], z = [phi_acc; theta_acc]
% CONVENTION:
%   * World = ENU, gravity = [0;0;-g]
%   * Body has +Z UP (thrust +bZ)
%   * acc_meas is IMU specific force in BODY (level: [0;0;+g])
% Units: rad, rad/s, m/s^2
%
% Added output:
%   K_gain : 4x2 Kalman gain used this step (zeros if accel update skipped)
%
%   State rows: [phi; theta; bp; bq]
%   Meas  cols: [phi_acc; theta_acc]
%   So, K_gain(1,1)=K_phi, K_gain(2,2)=K_theta,
%        K_gain(3,1)=K_bp_from_phi, K_gain(4,2)=K_bq_from_theta
%   Angles’ gains (how much the accel tilt corrects the angles) are: 𝐾𝜙=K_11 (row 1, col 1) 𝐾𝜃=K_22 (row 2, col 2) 
%   Bias gains (how much tilt corrects gyro biases): K bp ​ =K_31, K bq ​ =K_42


% ------- Axis sign switches (match EKF axes to your plant) -------
% +1 = same direction as plant; -1 = flip.
sX = 1;   % roll axis sign
sY = 1;   % pitch axis sign
sZ = +1;  % yaw/acc Z sign (Z up: az ≈ +g)

persistent x P psi
if isempty(x) || reset
    x   = [0; 0; 0; 0];   % [phi; theta; bp; bq]
    P   = diag([deg2rad(5)^2, deg2rad(5)^2, 0.05^2, 0.05^2]);
    psi = 0;
end

% ---- Apply mapping to measurements ----
% Gyros (rad/s)
p = sX * pqr_meas(1);
q = sY * pqr_meas(2);
r = sZ * pqr_meas(3);
% Accels (m/s^2)
ax = sX * acc_meas(1);
ay = sY * acc_meas(2);
az = sZ * acc_meas(3);

% ---- State unpack ----
phi   = x(1); theta = x(2);
bp    = x(3); bq    = x(4);

% ---- Predict ----
phi_minus   = phi   + (p - bp)*dt;
theta_minus = theta + (q - bq)*dt;
bp_minus    = bp; bq_minus = bq;

x_minus = [phi_minus; theta_minus; bp_minus; bq_minus];

F = eye(4); F(1,3) = -dt; F(2,4) = -dt;
Q = diag([ (sigma_g^2)*dt^2, (sigma_g^2)*dt^2, (sigma_bw(1)^2)*dt, (sigma_bw(2)^2)*dt ]);
P_minus = F*P*F.' + Q;

% ---- Accelerometer tilt update (body-Z up & specific force) ----
g   = 9.80665;
den = hypot(ay, az);
mag = sqrt(ax*ax + ay*ay + az*az);
use_acc = (den > 1e-6) && (abs(mag - g) < 3.0);

H = [1 0 0 0;
     0 1 0 0];
R = diag([sigma_tilt^2, sigma_tilt^2]);

% Prepare gain output (zeros if no update)
K_gain = zeros(4,2);

if use_acc
    % Correct tilt formulas for body-Z up & specific force
    phi_acc   = atan2(+ay, +az);    % roll from y/z
    theta_acc = atan2(-ax,  den);   % pitch from x & |yz|
    z = [phi_acc; theta_acc];

    % Innovation & gain
    y = z - H*x_minus;
    S = H*P_minus*H.' + R;
    K = (P_minus*H.')/S;

    % Update
    x = x_minus + K*y;
    P = (eye(4) - K*H)*P_minus;

    % Expose K
    K_gain = K;
else
    x = x_minus;
    P = P_minus;
end

% ---- Yaw dead-reckon ----
psi = psi + r*dt;

% ---- Outputs ----
eul_hat = [x(1); x(2); psi];
b_hat   = [x(3); x(4); 0];

end

== matlab function Quad_PID_attack_done/Attitude Dynamics/MATLAB Function4 ==
  data: roll_ddot output; torque input; euler_dot input; pitch_ddot output; yaw_ddot output; disturbance_torque input
function [roll_ddot, pitch_ddot, yaw_ddot] = Attitude_Dynamics(torque,euler_dot,disturbance_torque)


roll_ddot  = 0;
pitch_ddot = 0;
yaw_ddot = 0;

Quad_Model.Ixx = 0.016;
Quad_Model.Iyy = 0.016;
Quad_Model.Izz = 0.0274;
Quad_Model.Im = 3.789*1e-6;  

roll_ddot  =  disturbance_torque(1) + euler_dot(2) *  euler_dot(3) * (Quad_Model.Iyy - Quad_Model.Izz) / Quad_Model.Ixx - Quad_Model.Im *  euler_dot(2) * 10 + torque(1) / Quad_Model.Ixx;
pitch_ddot =  disturbance_torque(2) + euler_dot(1) *  euler_dot(3) * (Quad_Model.Izz - Quad_Model.Ixx) / Quad_Model.Iyy + Quad_Model.Im *  euler_dot(1) * 10 + torque(2) / Quad_Model.Iyy;
yaw_ddot   =  disturbance_torque(3) + euler_dot(1) *  euler_dot(2) * (Quad_Model.Ixx - Quad_Model.Iyy) / Quad_Model.Izz + torque(3) / Quad_Model.Izz;



end

== matlab function Quad_PID_attack_done/Position Dynamics/MATLAB Function5 ==
  data: acc_x output; euler input; thrust input; disturbance input; acc_y output; acc_z output
function [acc_x,acc_y,acc_z] = Position_Dynamics(euler,thrust,disturbance)
Quad_Model.mass = 1;
Quad_Model.g = 9.8;

acc_x = 0;
acc_y = 0;
acc_z = 0;

acc_x = disturbance(1) + (cos(euler(1)) * sin(euler(2)) * cos(euler(3)) + sin(euler(1)) * sin(euler(3))) * thrust / Quad_Model.mass;
acc_y = disturbance(2) + (cos(euler(1)) * sin(euler(2)) * sin(euler(3)) - sin(euler(1)) * cos(euler(3))) * thrust / Quad_Model.mass;
acc_z = disturbance(3) - Quad_Model.g + cos(euler(1)) * cos(euler(2)) * thrust / Quad_Model.mass;    

end
